simulink model "Eq7_CyclesLoss"  (R2022b)
settings: Solver=FixedStepAuto  StartTime=0.0  StopTime=10.0  RelTol=1e-3
settings Model: Creator=umber  LastModifiedBy=umber
settings OptimizationCC: OptimizeBlockIOStorage=off  OptimizeDataStoreBuffers=off  BusAssignmentInplaceUpdate=off
settings DebuggingCC: SFUnexpectedBacktrackingDiag=warning  SFNoUnconditionalDefaultTransitionDiag=warning
settings ModelReferenceCC: EnableRefExpFcnMdlSchedulingChecks=on
settings RTWCC: GenerateReport=on  BuildConfiguration=Debug  LaunchReport=on
settings CodeAppCC: ForceParamTrailComments=on  MATLABSourceComments=on  EnableCustomComments=on
settings GRTTargetCC: CombineSignalStateStructs=on  SupportVariableSizeSignals=on  MultiInstanceErrorCode=Warning

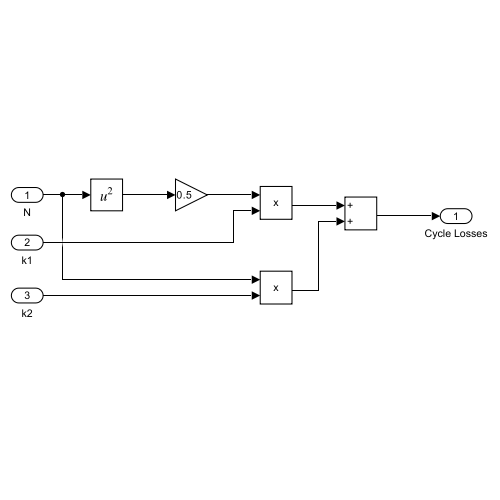
[thumbnail: Simulink's stored preview of the top-level diagram]
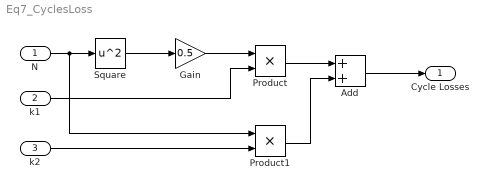
== system Eq7_CyclesLoss ==
  N : Inport
  k1 : Inport  Port=2
  k2 : Inport  Port=3
  Add : Sum
  Gain : Gain  Gain=0.5
  Product : Product
  Product1 : Product
  Square : Math  Operator=square
  Cycle Losses : Outport
  wires:
  N/1 -> Product1/1, Square/1
  Square/1 -> Gain/1
  k1/1 -> Product/2
  Gain/1 -> Product/1
  Add/1 -> Cycle Losses/1
  Product/1 -> Add/1
  k2/1 -> Product1/2
  Product1/1 -> Add/2
